simulink model "Lab02_Part2"  (R2017b)
settings: Solver=VariableStepAuto  StartTime=0.0  StopTime=tf  MaxStep=maxstep  RelTol=tol  AbsTol=tol
values from neighbouring files (symbols this model uses):
  b = 1    [Lab2Script.m]    (also in Lab2Script_class.m)
  f = 10    [Lab2Script.m]    (also in Lab2Script_class.m)
  m = 2    [Lab2Script.m]    (also in Lab2Script_class.m = 1)
  v0 = 5    [Lab2Script.m]    (also in Lab2Script_class.m = 0)
settings Model: Creator=rodrigue  LastModifiedBy=rodrigue

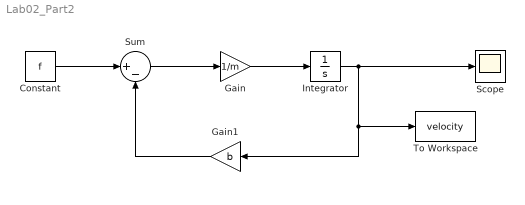
== system Lab02_Part2 ==
  Constant : Constant  Value=f
  Gain : Gain  Gain=1/m
  Gain1 : Gain  Gain=b
  Integrator : Integrator  InitialCondition=v0
  Scope : Scope
  Sum : Sum  Inputs=|+-
  To Workspace : ToWorkspace  VariableName=velocity  SampleTime=-1
  wires:
  Constant/1 -> Sum/1
  Sum/1 -> Gain/1
  Gain/1 -> Integrator/1
  Gain1/1 -> Sum/2
  Integrator/1 -> To Workspace/1, Gain1/1, Scope/1
